simulink model "three_levelparallel_spwm"  (R2016a)
settings: Solver=VariableStepAuto  StartTime=0.0  StopTime=stop_time  RelTol=1e-3
undefined symbols (not defined in the file): DCLINK_Cap1, DCLINK_Cap2, interleaving_angle, Lload, ma, ref_frequency, Rload, Sampling_time, Vin
libraries: powerlib x65, simulink x12, powerlib_meascontrol x10
settings Model: Creator=hakan  LastModifiedBy=hakan
settings DataIOCC: LimitDataPoints=on
settings DebuggingCC: AllowSymbolicDim=off
settings ModelReferenceCC: PropagateSignalLabelsOutOfModel=off
settings GRTTargetCC: GeneratePreprocessorConditionals=Use local settings

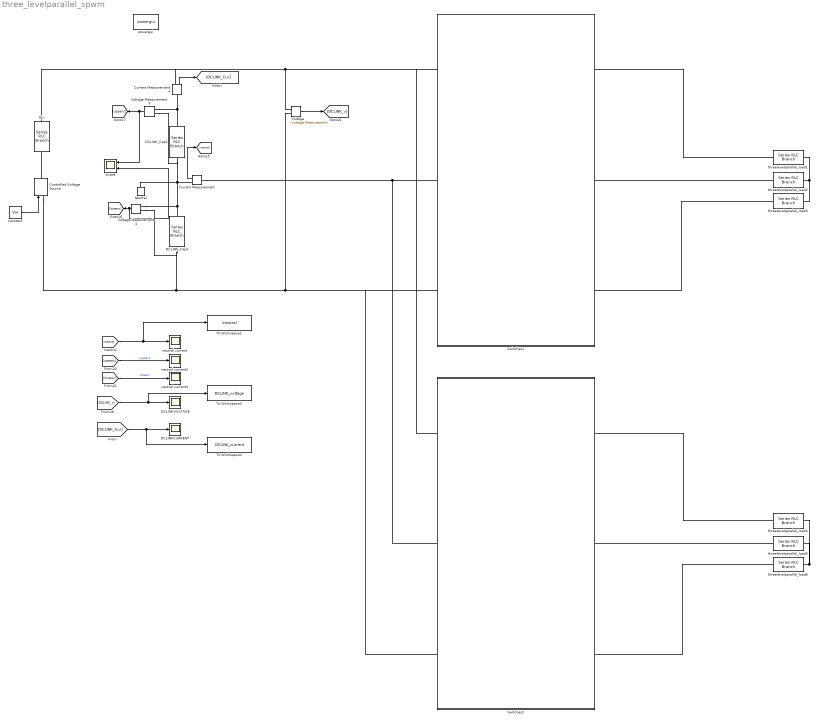
== system three_levelparallel_spwm ==
  Constant : Constant  Value=Vin
  Controlled Voltage Source : powerlib/Electrical Sources/Controlled Voltage Source  Initialize=on  Source_Type=AC  Amplitude=0  Phase=0  Frequency=0  Measurements=None
  Current Measurement : powerlib/Measurements/Current Measurement  PhasorSimulation=off  OutputType=Complex  PSBequivalent=0
  Current Measurement4 : powerlib/Measurements/Current Measurement  PhasorSimulation=off  OutputType=Complex  PSBequivalent=0
  DCLINKCURRENT : Scope
  DCLINKVOLTAGE : Scope
  DCLINK_Cap1 : powerlib/Elements/Series RLC Branch  LConnTagsString=__new0  RConnTagsString=__new0  BranchType=C  Resistance=1  Inductance=1e-3  SetiL0=off  InitialCurrent=0  Capacitance=DCLINK_Cap1  Setx0=off  InitialVoltage=0  Measurements=None
  DCLINK_Cap2 : powerlib/Elements/Series RLC Branch  LConnTagsString=__new0  RConnTagsString=__new0  BranchType=C  Resistance=1  Inductance=1e-3  SetiL0=off  InitialCurrent=0  Capacitance=DCLINK_Cap2  Setx0=off  InitialVoltage=0  Measurements=None
  Neutral : powerlib/Elements/Neutral  LConnTagsString=a  NodeNumber=10
  Rin : powerlib/Elements/Series RLC Branch  LConnTagsString=__new0  RConnTagsString=__new0  BranchType=R  Resistance=1  Inductance=1e-3  SetiL0=off  InitialCurrent=0  Capacitance=1000e-6  Setx0=off  InitialVoltage=0  Measurements=None
  Scope : Scope  NumInputPorts=2
  Switches1 : Subsystem
  Switches2 : Subsystem
  To Workspace1 : ToWorkspace  VariableName=Ineutral  SaveFormat=Timeseries  SampleTime=-1
  To Workspace3 : ToWorkspace  VariableName=DCLINK_voltage  SaveFormat=Timeseries  SampleTime=-1
  To Workspace4 : ToWorkspace  VariableName=DCLINK_current  SaveFormat=Timeseries  SampleTime=-1
  "Voltage " : powerlib/Measurements/Voltage Measurement  PhasorSimulation=off  OutputType=Complex  PSBequivalent=0
  Voltage Measurement3 : powerlib/Measurements/Voltage Measurement  PhasorSimulation=off  OutputType=Complex  PSBequivalent=0
  Voltage Measurement4 : powerlib/Measurements/Voltage Measurement  PhasorSimulation=off  OutputType=Complex  PSBequivalent=0
  neutral current : Scope
  neutral current2 : Scope
  neutral current3 : Scope
  powergui : powerlib/powergui  Priority=1  SimulationMode=Discrete  SolverType=Tustin/Backward Euler (TBE)  SampleTime=Sampling_time  frequency=60  SPID=off  DisableSnubberDevices=off  DisableRonSwitches=off  DisableVfSwitches=off  SwTol=0  DisplayEquations=off  Interpol=off  ExternalGateDelay=off  methode=off  Ts=10  FunctionMessages=off  echomessages=off  HookPort=off  EnableUseOfTLC=off  x0status=blocks  frequencyindice=0  Pbase=100e6  ErrMax=1e-4  Iterations=50  UnitsV=kV  UnitsW=MW  buscounter=0  RestoreLinks=warning  ResistiveCurrentMeasurement=off  Frange=[0:2:500]  Ylog=off  Xlog=on  ShowGrid=off  save=off  variable=ZData  structure=Cap_V_One  ZoomFFT=off  StartTime=3  cycles=50  DisplayStyle=2  fundamental=50  FreqAxis=off  MaxFrequency=2000  frequencyindicesteady=1  RmsSteady=1  display=off
  threelevelparallel_load{1..6} (6 alike) : powerlib/Elements/Series RLC Branch  LConnTagsString=__new0  RConnTagsString=__new0  BranchType=RL  Resistance=Rload  Inductance=Lload  SetiL0=off  InitialCurrent=0  Capacitance=1e-6  Setx0=off  InitialVoltage=0  Measurements=None
  wires:
  Voltage Measurement3/1 -> Scope/1, [upperc]
  Voltage Measurement4/1 -> Scope/2, [lowerc]
  Current Measurement/1 -> [Ineutral]
  [Ineutral] -> To Workspace1/1, neutral current/1
  [lowerc] -> neutral current3/1  "lowerc"
  [upperc] -> neutral current2/1  "upperc"
  "Voltage "/1 -> [DCLINK_v]
  [DCLINK_v] -> To Workspace3/1, DCLINKVOLTAGE/1
  Current Measurement4/1 -> [DCLINK_Cur]
  [DCLINK_Cur] -> DCLINKCURRENT/1, To Workspace4/1
  Constant/1 -> Controlled Voltage Source/1
  connections:
  DCLINK_Cap2/RConn1 -- Voltage Measurement4/LConn2 -- Controlled Voltage Source/LConn1 -- Switches2/LConn3 -- Switches1/LConn3 -- "Voltage "/LConn2
  Voltage Measurement4/LConn1 -- Neutral/LConn1 -- DCLINK_Cap1/RConn1 -- Voltage Measurement3/LConn2 -- Current Measurement/RConn1 -- DCLINK_Cap2/LConn1
  "Voltage "/LConn1 -- Switches2/LConn1 -- Switches1/LConn1 -- Rin/LConn1 -- Current Measurement4/RConn1
  Switches1/RConn1 -- threelevelparallel_load1/LConn1
  Current Measurement/LConn1 -- Switches2/LConn2 -- Switches1/LConn2
  threelevelparallel_load2/LConn1 -- Switches1/RConn2
  Switches1/RConn3 -- threelevelparallel_load3/LConn1
  Voltage Measurement3/LConn1 -- Current Measurement4/LConn1 -- DCLINK_Cap1/LConn1
  threelevelparallel_load5/LConn1 -- Switches2/RConn2
  Switches2/RConn3 -- threelevelparallel_load6/LConn1
  Switches2/RConn1 -- threelevelparallel_load4/LConn1
  threelevelparallel_load1/RConn1 -- threelevelparallel_load3/RConn1 -- threelevelparallel_load2/RConn1
  threelevelparallel_load6/RConn1 -- threelevelparallel_load4/RConn1 -- threelevelparallel_load5/RConn1
  Controlled Voltage Source/RConn1 -- Rin/RConn1

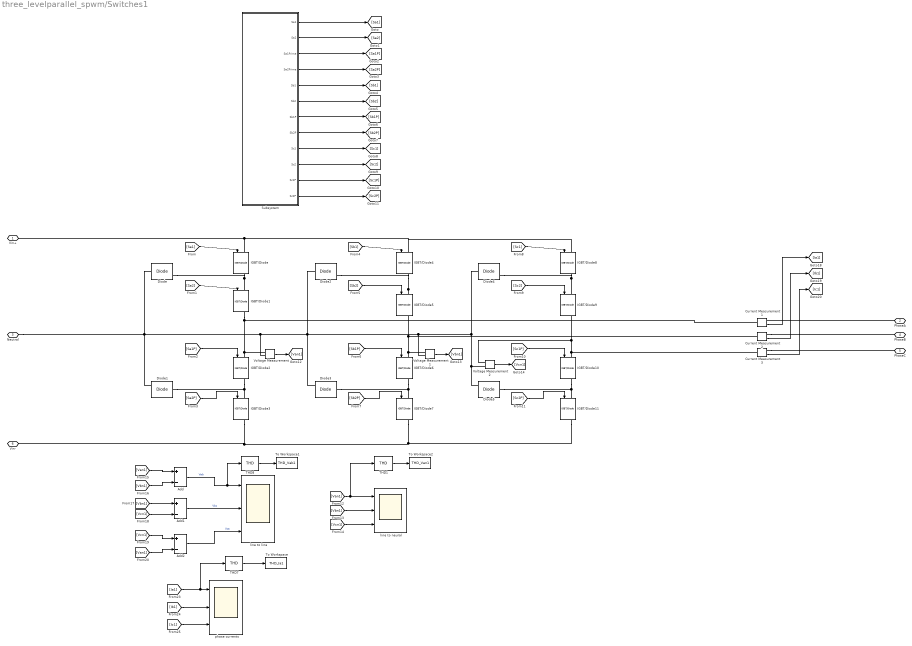
== system three_levelparallel_spwm/Switches1 ==
  Add : Sum  Inputs=+-
  Add1 : Sum  Inputs=+-
  Add2 : Sum  Inputs=+-
  Current Measurement1 : powerlib/Measurements/Current Measurement  PhasorSimulation=off  OutputType=Complex  PSBequivalent=0
  Current Measurement2 : powerlib/Measurements/Current Measurement  PhasorSimulation=off  OutputType=Complex  PSBequivalent=0
  Current Measurement3 : powerlib/Measurements/Current Measurement  PhasorSimulation=off  OutputType=Complex  PSBequivalent=0
  Diode{,1..5} (6 alike) : powerlib/Power Electronics/Diode  Ron=0.001  Lon=0  Vf=0.8  IC=0  UseSnubber=off  Rs=500  Cs=250e-9  Measurements=on
  IGBT/Diode{,1..11} (12 alike) : powerlib/Power Electronics/IGBT//Diode  Ron=1e-3  Rs=1e5  Cs=inf  Measurements=on
  Subsystem : Subsystem
  THD1 : powerlib_meascontrol/Measurements/THD  Freq=50  Ts=0
  THD7 : powerlib_meascontrol/Measurements/THD  Freq=50  Ts=0
  THD8 : powerlib_meascontrol/Measurements/THD  Freq=50  Ts=0
  To Workspace : ToWorkspace  VariableName=THD_Ia1  SaveFormat=Timeseries  SampleTime=-1
  To Workspace1 : ToWorkspace  VariableName=THD_Vab1  SaveFormat=Timeseries  SampleTime=-1
  To Workspace2 : ToWorkspace  VariableName=THD_Van1  SaveFormat=Timeseries  SampleTime=-1
  Voltage Measurement : powerlib/Measurements/Voltage Measurement  PhasorSimulation=off  OutputType=Complex  PSBequivalent=0
  Voltage Measurement1 : powerlib/Measurements/Voltage Measurement  PhasorSimulation=off  OutputType=Complex  PSBequivalent=0
  Voltage Measurement2 : powerlib/Measurements/Voltage Measurement  PhasorSimulation=off  OutputType=Complex  PSBequivalent=0
  line to line : Scope  NumInputPorts=3
  line to neural : Scope  NumInputPorts=3
  phase currents : Scope  NumInputPorts=3
  Vin+ : PMIOPort  Port=1  Side=Left
  "PhaseA " : PMIOPort  Port=2  Side=Right
  Neutral : PMIOPort  Port=3  Side=Left
  PhaseB : PMIOPort  Port=4  Side=Right
  PhaseC : PMIOPort  Port=5  Side=Right
  Vin- : PMIOPort  Port=6  Side=Left
  wires:
  [Sa1] -> IGBT/Diode/1
  [Sa2] -> IGBT/Diode1/1
  Subsystem/4("Sa2Prime ") -> [Sa2P]
  Subsystem/1("Sa1 ") -> [Sa1]
  Subsystem/2("Sa2 ") -> [Sa2]
  Subsystem/3(Sa1Prime) -> [Sa1P]
  Subsystem/6(Sb2) -> [Sb2]
  [Sa2P] -> IGBT/Diode3/1
  [Sc2P] -> IGBT/Diode11/1
  [Sc1] -> IGBT/Diode8/1
  [Sc1P] -> IGBT/Diode10/1
  Subsystem/8(Sb2P) -> [Sb2P]
  Subsystem/9("Sc1 ") -> [Sc1]
  [Sa1P] -> IGBT/Diode2/1
  Subsystem/12("Sc2P ") -> [Sc2P]
  Voltage Measurement1/1 -> [Vbn1]
  [Sb1P] -> IGBT/Diode6/1
  Subsystem/10(Sc2) -> [Sc2]
  Subsystem/11(Sc1P) -> [Sc1P]
  Voltage Measurement2/1 -> [Vcn1]
  [Van1] -> Add/1
  [Sb2P] -> IGBT/Diode7/1
  [Vbn1] -> Add/2
  [Sb1] -> IGBT/Diode4/1
  [Sc2] -> IGBT/Diode9/1
  Subsystem/5(Sb1) -> [Sb1]
  Subsystem/7("Sb1P ") -> [Sb1P]
  [Sb2] -> IGBT/Diode5/1
  Voltage Measurement/1 -> [Van1]
  [Van1] -> THD1/1, line to neural/1
  [Vbn1] -> line to neural/2
  Add/1 -> THD8/1, line to line/1  "Vab"
  [Vcn1] -> Add2/1
  [Vcn1] -> line to neural/3
  [Ib1] -> phase currents/2
  [Vbn1] -> Add1/1
  Add2/1 -> line to line/3  "Vca"
  [Van1] -> Add2/2
  Add1/1 -> line to line/2  "Vbc"
  [Ic1] -> phase currents/3
  [Vcn1] -> Add1/2
  THD7/1 -> To Workspace/1
  [Ia1] -> THD7/1, phase currents/1
  THD8/1 -> To Workspace1/1
  THD1/1 -> To Workspace2/1
  Current Measurement1/1 -> [Ia1]
  Current Measurement2/1 -> [Ib1]
  Current Measurement3/1 -> [Ic1]
  connections:
  IGBT/Diode/RConn1 -- Diode/RConn1 -- IGBT/Diode1/LConn1
  IGBT/Diode8/LConn1 -- IGBT/Diode4/LConn1 -- Vin+/RConn1 -- IGBT/Diode/LConn1
  IGBT/Diode1/RConn1 -- Current Measurement1/LConn1 -- Voltage Measurement/LConn1 -- IGBT/Diode2/LConn1
  IGBT/Diode2/RConn1 -- Diode1/LConn1 -- IGBT/Diode3/LConn1
  Diode5/LConn1 -- IGBT/Diode11/LConn1 -- IGBT/Diode10/RConn1
  IGBT/Diode5/LConn1 -- Diode2/RConn1 -- IGBT/Diode4/RConn1
  Diode4/RConn1 -- IGBT/Diode8/RConn1 -- IGBT/Diode9/LConn1
  IGBT/Diode6/RConn1 -- Diode3/LConn1 -- IGBT/Diode7/LConn1
  IGBT/Diode9/RConn1 -- Voltage Measurement2/LConn1 -- Current Measurement3/LConn1 -- IGBT/Diode10/LConn1
  IGBT/Diode5/RConn1 -- Voltage Measurement1/LConn1 -- IGBT/Diode6/LConn1 -- Current Measurement2/LConn1
  Diode5/RConn1 -- Voltage Measurement2/LConn2 -- Diode4/LConn1 -- Voltage Measurement1/LConn2 -- Diode3/RConn1 -- Voltage Measurement/LConn2 -- Diode1/RConn1 -- Neutral/RConn1 -- Diode/LConn1 -- Diode2/LConn1
  IGBT/Diode11/RConn1 -- Vin-/RConn1 -- IGBT/Diode3/RConn1 -- IGBT/Diode7/RConn1
  "PhaseA "/RConn1 -- Current Measurement1/RConn1
  Current Measurement2/RConn1 -- PhaseB/RConn1
  Current Measurement3/RConn1 -- PhaseC/RConn1

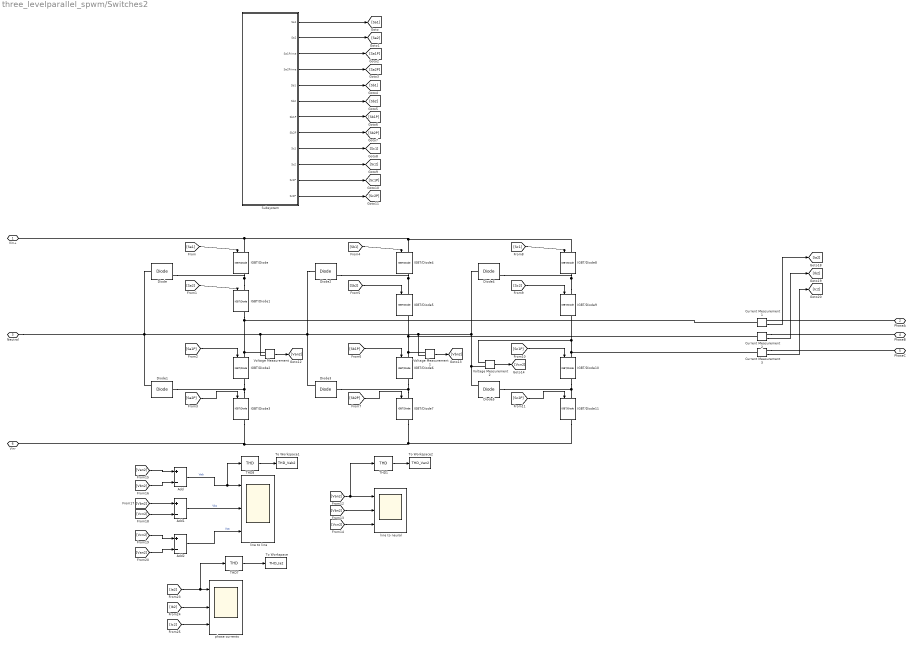
== system three_levelparallel_spwm/Switches2 ==
  Add : Sum  Inputs=+-
  Add1 : Sum  Inputs=+-
  Add2 : Sum  Inputs=+-
  Current Measurement1 : powerlib/Measurements/Current Measurement  PhasorSimulation=off  OutputType=Complex  PSBequivalent=0
  Current Measurement2 : powerlib/Measurements/Current Measurement  PhasorSimulation=off  OutputType=Complex  PSBequivalent=0
  Current Measurement3 : powerlib/Measurements/Current Measurement  PhasorSimulation=off  OutputType=Complex  PSBequivalent=0
  Diode{,1..5} (6 alike) : powerlib/Power Electronics/Diode  Ron=0.001  Lon=0  Vf=0.8  IC=0  UseSnubber=off  Rs=500  Cs=250e-9  Measurements=on
  IGBT/Diode{,1..11} (12 alike) : powerlib/Power Electronics/IGBT//Diode  Ron=1e-3  Rs=1e5  Cs=inf  Measurements=on
  Subsystem : Subsystem
  THD1 : powerlib_meascontrol/Measurements/THD  Freq=50  Ts=0
  THD7 : powerlib_meascontrol/Measurements/THD  Freq=50  Ts=0
  THD8 : powerlib_meascontrol/Measurements/THD  Freq=50  Ts=0
  To Workspace : ToWorkspace  VariableName=THD_Ia2  SaveFormat=Timeseries  SampleTime=-1
  To Workspace1 : ToWorkspace  VariableName=THD_Vab2  SaveFormat=Timeseries  SampleTime=-1
  To Workspace2 : ToWorkspace  VariableName=THD_Van2  SaveFormat=Timeseries  SampleTime=-1
  Voltage Measurement : powerlib/Measurements/Voltage Measurement  PhasorSimulation=off  OutputType=Complex  PSBequivalent=0
  Voltage Measurement1 : powerlib/Measurements/Voltage Measurement  PhasorSimulation=off  OutputType=Complex  PSBequivalent=0
  Voltage Measurement2 : powerlib/Measurements/Voltage Measurement  PhasorSimulation=off  OutputType=Complex  PSBequivalent=0
  line to line : Scope  NumInputPorts=3
  line to neural : Scope  NumInputPorts=3
  phase currents : Scope  NumInputPorts=3
  Vin+ : PMIOPort  Port=1  Side=Left
  "PhaseA " : PMIOPort  Port=2  Side=Right
  Neutral : PMIOPort  Port=3  Side=Left
  PhaseB : PMIOPort  Port=4  Side=Right
  PhaseC : PMIOPort  Port=5  Side=Right
  Vin- : PMIOPort  Port=6  Side=Left
  wires:
  Current Measurement3/1 -> [Ic2]
  Current Measurement2/1 -> [Ib2]
  Current Measurement1/1 -> [Ia2]
  THD1/1 -> To Workspace2/1
  THD8/1 -> To Workspace1/1
  [Ia2] -> phase currents/1, THD7/1
  THD7/1 -> To Workspace/1
  [Vcn2] -> Add1/2
  [Ic2] -> phase currents/3
  Add1/1 -> line to line/2  "Vbc"
  [Van2] -> Add2/2
  Add2/1 -> line to line/3  "Vca"
  [Vbn2] -> Add1/1
  [Ib2] -> phase currents/2
  [Vcn2] -> line to neural/3
  [Vcn2] -> Add2/1
  Add/1 -> line to line/1, THD8/1  "Vab"
  [Vbn2] -> line to neural/2
  [Van2] -> line to neural/1, THD1/1
  Voltage Measurement/1 -> [Van2]
  [Sb2] -> IGBT/Diode5/1
  Subsystem/7("Sb1P ") -> [Sb1P]
  Subsystem/5(Sb1) -> [Sb1]
  [Sc2] -> IGBT/Diode9/1
  [Sb1] -> IGBT/Diode4/1
  [Vbn2] -> Add/2
  [Sb2P] -> IGBT/Diode7/1
  [Van2] -> Add/1
  Voltage Measurement2/1 -> [Vcn2]
  Subsystem/11(Sc1P) -> [Sc1P]
  Subsystem/10(Sc2) -> [Sc2]
  [Sb1P] -> IGBT/Diode6/1
  Voltage Measurement1/1 -> [Vbn2]
  Subsystem/12("Sc2P ") -> [Sc2P]
  [Sa1P] -> IGBT/Diode2/1
  Subsystem/9("Sc1 ") -> [Sc1]
  Subsystem/8(Sb2P) -> [Sb2P]
  [Sc1P] -> IGBT/Diode10/1
  [Sc1] -> IGBT/Diode8/1
  [Sc2P] -> IGBT/Diode11/1
  [Sa2P] -> IGBT/Diode3/1
  Subsystem/6(Sb2) -> [Sb2]
  Subsystem/3(Sa1Prime) -> [Sa1P]
  Subsystem/2("Sa2 ") -> [Sa2]
  Subsystem/1("Sa1 ") -> [Sa1]
  Subsystem/4("Sa2Prime ") -> [Sa2P]
  [Sa2] -> IGBT/Diode1/1
  [Sa1] -> IGBT/Diode/1
  connections:
  Current Measurement3/RConn1 -- PhaseC/RConn1
  Current Measurement2/RConn1 -- PhaseB/RConn1
  "PhaseA "/RConn1 -- Current Measurement1/RConn1
  IGBT/Diode7/RConn1 -- IGBT/Diode3/RConn1 -- Vin-/RConn1 -- IGBT/Diode11/RConn1
  Diode2/LConn1 -- Diode/LConn1 -- Neutral/RConn1 -- Diode1/RConn1 -- Voltage Measurement/LConn2 -- Diode3/RConn1 -- Voltage Measurement1/LConn2 -- Diode4/LConn1 -- Voltage Measurement2/LConn2 -- Diode5/RConn1
  Current Measurement2/LConn1 -- IGBT/Diode6/LConn1 -- Voltage Measurement1/LConn1 -- IGBT/Diode5/RConn1
  IGBT/Diode10/LConn1 -- Current Measurement3/LConn1 -- Voltage Measurement2/LConn1 -- IGBT/Diode9/RConn1
  IGBT/Diode7/LConn1 -- Diode3/LConn1 -- IGBT/Diode6/RConn1
  IGBT/Diode9/LConn1 -- IGBT/Diode8/RConn1 -- Diode4/RConn1
  IGBT/Diode4/RConn1 -- Diode2/RConn1 -- IGBT/Diode5/LConn1
  IGBT/Diode10/RConn1 -- IGBT/Diode11/LConn1 -- Diode5/LConn1
  IGBT/Diode3/LConn1 -- Diode1/LConn1 -- IGBT/Diode2/RConn1
  IGBT/Diode2/LConn1 -- Voltage Measurement/LConn1 -- Current Measurement1/LConn1 -- IGBT/Diode1/RConn1
  IGBT/Diode/LConn1 -- Vin+/RConn1 -- IGBT/Diode4/LConn1 -- IGBT/Diode8/LConn1
  IGBT/Diode1/LConn1 -- Diode/RConn1 -- IGBT/Diode/RConn1

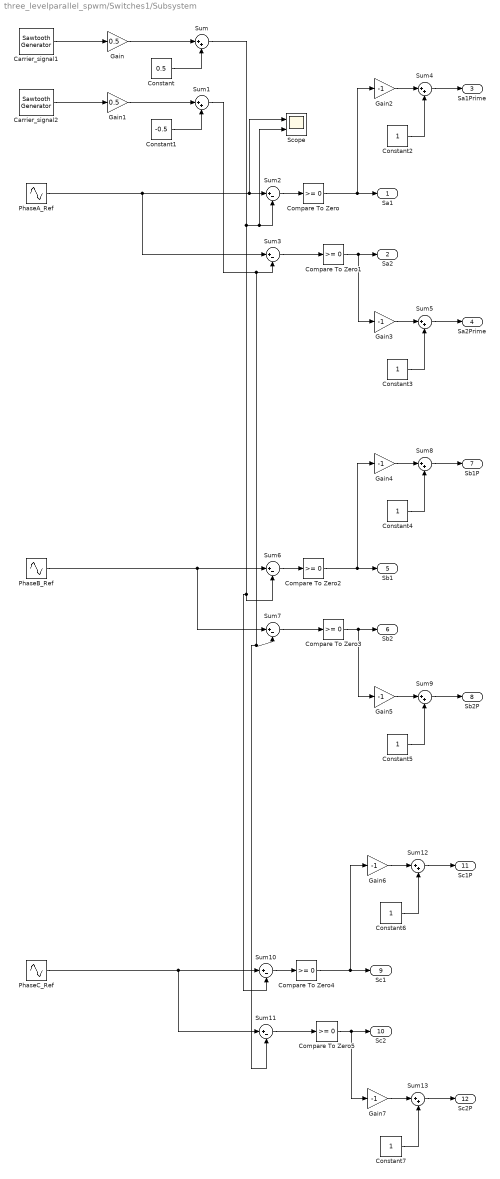
== system three_levelparallel_spwm/Switches1/Subsystem ==
  Carrier_signal1 : powerlib_meascontrol/Pulse & Signal Generators/Sawtooth Generator  Freq=sw_frequency  Phase=0  Ts=0
  Carrier_signal2 : powerlib_meascontrol/Pulse & Signal Generators/Sawtooth Generator  Freq=sw_frequency  Phase=0  Ts=0
  Compare To Zero{,1..5} (6 alike) : simulink/Logic and Bit Operations/Compare To Zero  relop=>=  OutDataTypeStr=boolean
  Constant : Constant  Value=0.5
  Constant1 : Constant  Value=-0.5
  Constant{2..7} (6 alike) : Constant
  Gain : Gain  Gain=0.5
  Gain1 : Gain  Gain=0.5
  Gain{2..7} (6 alike) : Gain  Gain=-1
  PhaseA_Ref : Sin  Amplitude=ma  Frequency=ref_frequency  SampleTime=0
  PhaseB_Ref : Sin  Amplitude=ma  Frequency=ref_frequency  Phase=2*pi/3  SampleTime=0
  PhaseC_Ref : Sin  Amplitude=ma  Frequency=ref_frequency  Phase=4*pi/3  SampleTime=0
  Scope : Scope  NumInputPorts=2
  Sum{,1,4..5,8..9,12..13} (8 alike) : Sum  Inputs=|++
  Sum{2..3,6..7,10..11} (6 alike) : Sum  Inputs=|+-
  "Sa1 " : Outport
  "Sa2 " : Outport  Port=2
  Sa1Prime : Outport  Port=3
  "Sa2Prime " : Outport  Port=4
  Sb1 : Outport  Port=5
  Sb2 : Outport  Port=6
  "Sb1P " : Outport  Port=7
  Sb2P : Outport  Port=8
  "Sc1 " : Outport  Port=9
  Sc2 : Outport  Port=10
  Sc1P : Outport  Port=11
  "Sc2P " : Outport  Port=12
  wires:
  Carrier_signal1/1 -> Gain/1
  Gain/1 -> Sum/1
  Sum/1 -> Scope/2, Sum2/2, Sum10/2, Sum6/2
  Constant/1 -> Sum/2
  Carrier_signal2/1 -> Gain1/1
  Gain1/1 -> Sum1/1
  Sum1/1 -> Sum11/2, Sum7/2, Sum3/2
  Constant1/1 -> Sum1/2
  PhaseA_Ref/1 -> Sum3/1, Scope/1, Sum2/1
  Sum2/1 -> Compare To Zero/1
  Compare To Zero/1 -> Gain2/1, "Sa1 "/1
  Sum3/1 -> Compare To Zero1/1
  Compare To Zero1/1 -> Gain3/1, "Sa2 "/1
  Constant2/1 -> Sum4/2
  Gain2/1 -> Sum4/1
  Sum4/1 -> Sa1Prime/1
  Constant3/1 -> Sum5/2
  Gain3/1 -> Sum5/1
  Sum5/1 -> "Sa2Prime "/1
  Sum6/1 -> Compare To Zero2/1
  Compare To Zero2/1 -> Sb1/1, Gain4/1
  Sum7/1 -> Compare To Zero3/1
  Compare To Zero3/1 -> Sb2/1, Gain5/1
  Constant4/1 -> Sum8/2
  Gain4/1 -> Sum8/1
  Sum8/1 -> "Sb1P "/1
  Constant5/1 -> Sum9/2
  Gain5/1 -> Sum9/1
  Sum9/1 -> Sb2P/1
  PhaseB_Ref/1 -> Sum7/1, Sum6/1
  Sum10/1 -> Compare To Zero4/1
  Compare To Zero4/1 -> Gain6/1, "Sc1 "/1
  Sum11/1 -> Compare To Zero5/1
  Compare To Zero5/1 -> Gain7/1, Sc2/1
  Constant6/1 -> Sum12/2
  Gain6/1 -> Sum12/1
  Sum12/1 -> Sc1P/1
  Constant7/1 -> Sum13/2
  Gain7/1 -> Sum13/1
  Sum13/1 -> "Sc2P "/1
  PhaseC_Ref/1 -> Sum11/1, Sum10/1

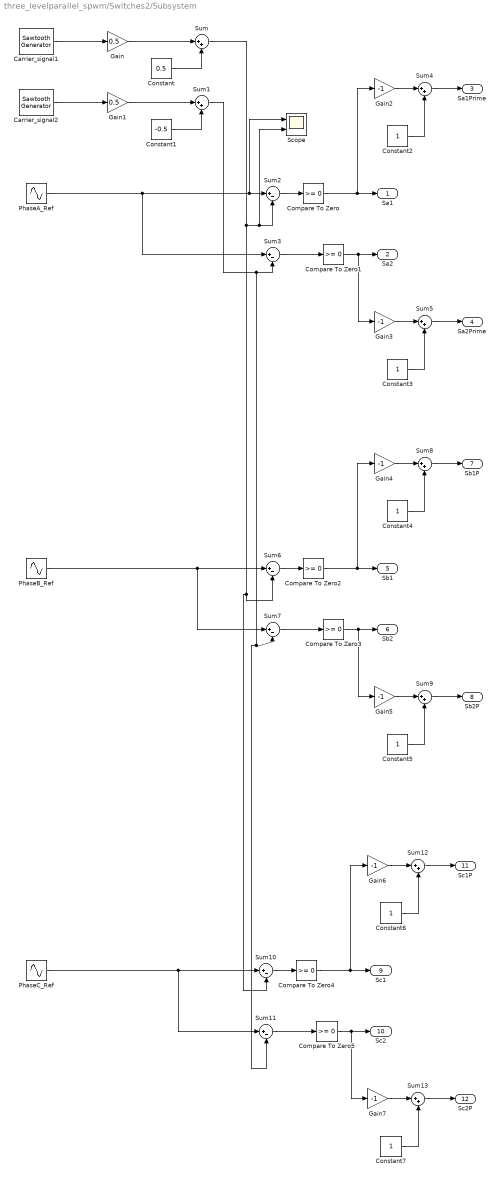
== system three_levelparallel_spwm/Switches2/Subsystem ==
  Carrier_signal1 : powerlib_meascontrol/Pulse & Signal Generators/Sawtooth Generator  Freq=sw_frequency  Phase=interleaving_angle  Ts=0
  Carrier_signal2 : powerlib_meascontrol/Pulse & Signal Generators/Sawtooth Generator  Freq=sw_frequency  Phase=interleaving_angle  Ts=0
  Compare To Zero{,1..5} (6 alike) : simulink/Logic and Bit Operations/Compare To Zero  relop=>=  OutDataTypeStr=boolean
  Constant : Constant  Value=0.5
  Constant1 : Constant  Value=-0.5
  Constant{2..7} (6 alike) : Constant
  Gain : Gain  Gain=0.5
  Gain1 : Gain  Gain=0.5
  Gain{2..7} (6 alike) : Gain  Gain=-1
  PhaseA_Ref : Sin  Amplitude=ma  Frequency=ref_frequency  SampleTime=0
  PhaseB_Ref : Sin  Amplitude=ma  Frequency=ref_frequency  Phase=2*pi/3  SampleTime=0
  PhaseC_Ref : Sin  Amplitude=ma  Frequency=ref_frequency  Phase=4*pi/3  SampleTime=0
  Scope : Scope  NumInputPorts=2
  Sum{,1,4..5,8..9,12..13} (8 alike) : Sum  Inputs=|++
  Sum{2..3,6..7,10..11} (6 alike) : Sum  Inputs=|+-
  "Sa1 " : Outport
  "Sa2 " : Outport  Port=2
  Sa1Prime : Outport  Port=3
  "Sa2Prime " : Outport  Port=4
  Sb1 : Outport  Port=5
  Sb2 : Outport  Port=6
  "Sb1P " : Outport  Port=7
  Sb2P : Outport  Port=8
  "Sc1 " : Outport  Port=9
  Sc2 : Outport  Port=10
  Sc1P : Outport  Port=11
  "Sc2P " : Outport  Port=12
  wires:
  PhaseC_Ref/1 -> Sum10/1, Sum11/1
  Sum13/1 -> "Sc2P "/1
  Gain7/1 -> Sum13/1
  Constant7/1 -> Sum13/2
  Sum12/1 -> Sc1P/1
  Gain6/1 -> Sum12/1
  Constant6/1 -> Sum12/2
  Compare To Zero5/1 -> Sc2/1, Gain7/1
  Sum11/1 -> Compare To Zero5/1
  Compare To Zero4/1 -> "Sc1 "/1, Gain6/1
  Sum10/1 -> Compare To Zero4/1
  PhaseB_Ref/1 -> Sum6/1, Sum7/1
  Sum9/1 -> Sb2P/1
  Gain5/1 -> Sum9/1
  Constant5/1 -> Sum9/2
  Sum8/1 -> "Sb1P "/1
  Gain4/1 -> Sum8/1
  Constant4/1 -> Sum8/2
  Compare To Zero3/1 -> Gain5/1, Sb2/1
  Sum7/1 -> Compare To Zero3/1
  Compare To Zero2/1 -> Gain4/1, Sb1/1
  Sum6/1 -> Compare To Zero2/1
  Sum5/1 -> "Sa2Prime "/1
  Gain3/1 -> Sum5/1
  Constant3/1 -> Sum5/2
  Sum4/1 -> Sa1Prime/1
  Gain2/1 -> Sum4/1
  Constant2/1 -> Sum4/2
  Compare To Zero1/1 -> "Sa2 "/1, Gain3/1
  Sum3/1 -> Compare To Zero1/1
  Compare To Zero/1 -> "Sa1 "/1, Gain2/1
  Sum2/1 -> Compare To Zero/1
  PhaseA_Ref/1 -> Sum2/1, Scope/1, Sum3/1
  Constant1/1 -> Sum1/2
  Sum1/1 -> Sum3/2, Sum7/2, Sum11/2
  Gain1/1 -> Sum1/1
  Carrier_signal2/1 -> Gain1/1
  Constant/1 -> Sum/2
  Sum/1 -> Sum6/2, Sum10/2, Sum2/2, Scope/2
  Gain/1 -> Sum/1
  Carrier_signal1/1 -> Gain/1
